simulink subsystem "DomesticLoadModel"  (R2021a)
settings: Solver=VariableStepAuto  StartTime=0.0  StopTime=10.0  RelTol=1e-3
libraries: spsVoltageMeasurementLib x2, spsControlledCurrentSourceLib x1
settings Model: Creator=Sajid Ali  LastModifiedBy=Sajid Ali

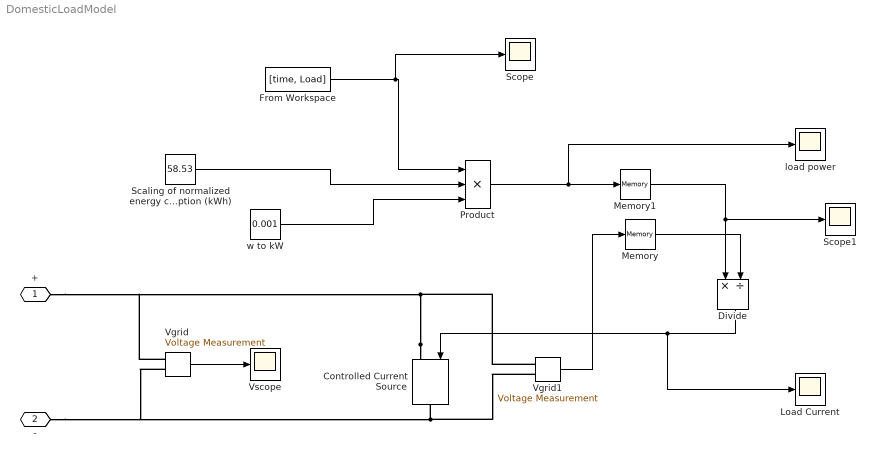
== system DomesticLoadModel ==
  Controlled Current Source : spsControlledCurrentSourceLib/Controlled Current Source  Initialize=on  Source_Type=DC  Amplitude=100  Phase=0  Frequency=50  Measurements=None
  Divide : Product  Inputs=*/
  From Workspace : FromWorkspace  VariableName=[time, Load]
  Load Current : Scope
  Memory : Memory  InitialCondition=100
  Memory1 : Memory  InitialCondition=2
  Product : Product  Inputs=3
  Scaling of normalized energy consumption (kWh) : Constant  Value=58.53
  Scope : Scope
  Scope1 : Scope
  Vgrid : spsVoltageMeasurementLib/Voltage Measurement  PhasorSimulation=off  OutputType=Complex  PSBequivalent=0
  Vgrid1 : spsVoltageMeasurementLib/Voltage Measurement  PhasorSimulation=off  OutputType=Complex  PSBequivalent=0
  Vscope : Scope
  load power : Scope
  w to kW : Constant  Value=0.001
  + : PMIOPort  Side=Left
  - : PMIOPort  Port=2  Side=Left
  wires:
  Vgrid/1 -> Vscope/1
  Divide/1 -> Load Current/1, Controlled Current Source/1
  Vgrid1/1 -> Memory/1
  Memory/1 -> Divide/2
  Product/1 -> load power/1, Memory1/1
  Memory1/1 -> Divide/1, Scope1/1
  w to kW/1 -> Product/3
  Scaling of normalized energy consumption (kWh)/1 -> Product/2
  From Workspace/1 -> Product/1, Scope/1
  connections:
  Controlled Current Source/LConn1 -- +/RConn1 -- Vgrid/LConn1 -- Vgrid1/LConn1
  Controlled Current Source/RConn1 -- Vgrid/LConn2 -- -/RConn1 -- Vgrid1/LConn2
